simulink model "project"  (R2017b)
settings: Solver=FixedStepDiscrete  StartTime=0.0  StopTime=inf  RelTol=1e-3
PreLoadFcn:
  | load('commwlan80211BusTypes')
PostLoadFcn:
  | commwlan80211BeaconModelParams('init')
InitFcn:
  | load('commwlan80211BusTypes')
model workspace: external: MAT-File (data not in the file)
undefined symbols (not defined in the file): commwlan80211TxFilt, p80211
libraries: commutil2 x6, commwlan80211BeaconLib x6, commcrc2 x3, commdigbbndpm3 x2, commsequence2 x2, commfilt2 x2, simulink x1, commsync2 x1, dspsigops x1, commchan3 x1, commrflib2 x1, commblksprivate x1
CloseFcn:
  | hFig = findall(0, 'Type', 'figure', 'Name', '802.11 Beacon Frame');
  | if ishghandle(hFig)
  | close(hFig);
  | end
  | clear hFig
Description:
  | IEEE 802.11 WLAN Beacon Frame
settings Model: Creator=The MathWorks, Inc.  LastModifiedBy=Josh Andrews
settings DataIOCC: LimitDataPoints=on  SaveFormat=Array  SaveOutput=off  SignalLogging=off  SaveTime=off
settings OptimizationCC: ExpressionDepthLimit=2147483647  LifeSpan=inf
settings DebuggingCC: UnderspecifiedInitializationDetection=Classic  MergeDetectMultiDrivingBlocksExec=none  SolverPrmCheckMsg=warning  FcnCallInpInsideContextMsg=warning  UniqueDataStoreMsg=error  AllowSymbolicDim=off  StateNameClashWarn=warning  SFUnexpectedBacktrackingDiag=warning  SFNoUnconditionalDefaultTransitionDiag=warning  SFExecutionAtInitializationDiag=none
settings HardwareCC: ProdBitPerPointer=32  ProdBitPerSizeT=32  ProdBitPerPtrDiffT=32  ProdLargestAtomicFloat=None  ProdIntDivRoundTo=Undefined  ProdEndianess=Unspecified  ProdWordSize=32  ProdHWDeviceType=32-bit Generic
settings ModelReferenceCC: PropagateSignalLabelsOutOfModel=off
settings CodeAppCC: StateflowObjectComments=on
settings GRTTargetCC: TargetLangStandard=C89/C90 (ANSI)  GeneratePreprocessorConditionals=Disable all  CombineOutputUpdateFcns=off  GRTInterface=on
settings ConfigComp: CovMetricSettings=dw  CovHtmlReporting=on  CovSaveCumulativeToWorkspaceVar=on  CovSaveSingleToWorkspaceVar=on  CovExternalEMLEnable=off  CovSFcnEnable=off

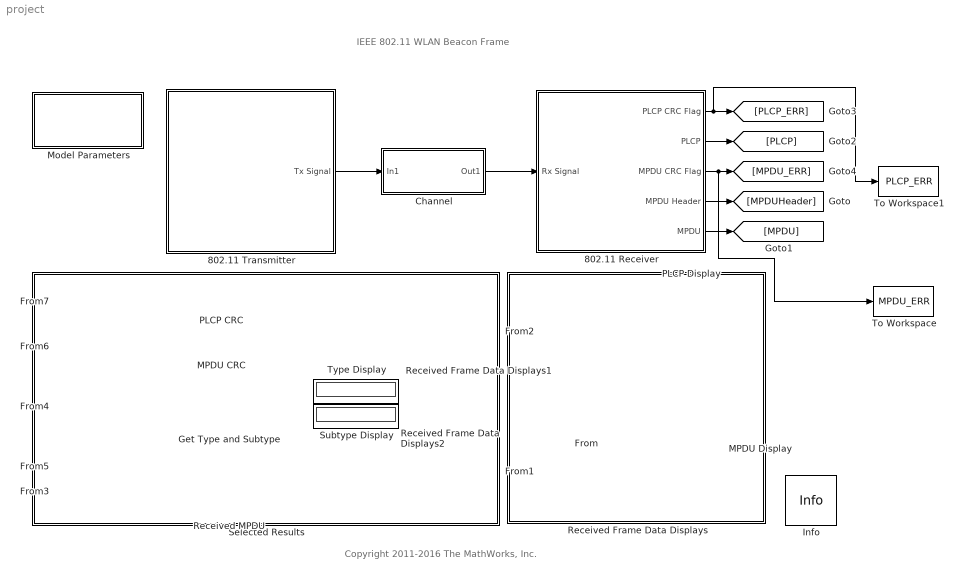
== system project ==
  note: IEEE 802.11 WLAN
      | Beacon Frame
  note: Copyright 2011-2016 The MathWorks, Inc.
  802.11 Receiver : Subsystem
  802.11 Transmitter : Subsystem
  Channel : Subsystem  BlockChoice=Delay only  mask(Channel){EsNo=0, freqOffset=100, delay=1e-06}
      mask prompts: EsNo "EsNo (dB):"; freqOffset "Frequency offset (Hz):"; delay "Delay (s):"
      mask help: Choose the channel type.
      settings: AttributesFormatString=Es/No = %<EsNo> dB\nFrequency offset = %<freqOffset> Hz\nDelay = %<delay> s
      mask Display: disp('Channel');
  Get Type and Subtype : Subsystem
  Info : commblksprivate/Info  SystemSampleTime=-1
      settings: SourceProductName=Communications System Toolbox  SourceProductBaseCode=CM
  MPDU CRC : Display
  MPDU Display : Subsystem
  Model Parameters : Subsystem  mask(Model Parameters){paramSet=Beacon frame parameters, beaconInterval=2, ssidValue='MathWorks SDR team', rates=[1 2 5], channelNumber=1, sendCFParams=on, cfpCount=2, cfpPeriod=5, cfpMaxDuration=10, cfpDurRemain=5, EsNo=0, freqOffset=100, delay=1e-6}
      mask prompts: paramSet "Parameter set:"; beaconInterval "Beacon interval (TU):"; ssidValue "SSID value:"; rates "Supported rates (Mbps):"; channelNumber "Channel number:"; sendCFParams "Send CF Parameters set element"; cfpCount "CFP Count (DTIM intervals):"; cfpPeriod "CFP Period (DTIM intervals):"; cfpMaxDuration "CFP MaxDuration (TU):"; cfpDurRemain "CFP DurRemaining (TU):"; EsNo "Es/No (dB):"; freqOffset "Frequency offset (Hz):"; delay "Delay (s):"
      mask help:
      | Choose beacon frame parameters and channel parameters.
      |
      | When you select the parameter set as 'Beacon frame parameters', you can set SSID, beacon interval, supported rates, channel number. You can also optionally send CF parameters set element in the beacon frame. The 'Beacon interval (TU)' parameter sets the period of beacon transmissions in time units (TU), which is 1024 microseconds.
      |
      | When you select the parameter set as 'Channel parameters', you can set noise level, frequency offset, and delay the channel introduces.
      mask init:
      | commwlan80211BeaconModelParams('init')
      settings: AttributesFormatString=Beacon interval = %<beaconInterval> TU
      mask Help: helpview(commdhelp);
      mask TypeOptions paramSet: Beacon frame parameters | Channel parameters
      mask Callback paramSet: commwlan80211BeaconModelParams('cbParamSet');
      mask TypeOptions channelNumber: 1 | 2 | 3 | 4 | 5 | 6 | 7 | 8 | 9 | 10 | 11
      mask Callback sendCFParams: commwlan80211BeaconModelParams('cbSendCFParams');
      mask Display: disp('Model\nParameters')
  PLCP CRC : Display
  PLCP Display : Subsystem
  Received Frame Data Displays : Subsystem
      mask Display: disp('')
  Received Frame Data Displays1 : Subsystem
      mask Display: disp('0 = Management')
  Received Frame Data Displays2 : Subsystem
      mask Display: disp('8 = Beacon')
  Received MPDU : Subsystem  mask(Received MPDU GUI){OpenScopeAtSimStart=on, openGUIBoolean=true}
      mask prompts: OpenScopeAtSimStart "Open GUI at start of simulation"; openGUIBoolean "Open GUI Boolean"
      mask help: Show selected information from the received Beacon frame.
      mask Callback OpenScopeAtSimStart:
      | if strcmp(get_param(gcb,'OpenScopeAtSimStart'), 'on')
      |   set_param(gcb,'openGUIBoolean','true');
      | else
      |   set_param(gcb,'openGUIBoolean','false');
      | end
      mask Display: disp('MPDU GUI')
  Selected Results : Subsystem
      mask Display: disp('')
  Subtype Display : Display
  To Workspace : ToWorkspace  VariableName=MPDU_ERR  SaveFormat=Timeseries  SampleTime=-1
  To Workspace1 : ToWorkspace  VariableName=PLCP_ERR  SaveFormat=Timeseries  SampleTime=-1
  Type Display : Display
  wires:
  Channel/1(Out1) -> 802.11 Receiver/1(Rx Signal)
  802.11 Receiver/1(PLCP CRC Flag) -> To Workspace1/1, [PLCP_ERR]
  802.11 Receiver/3(MPDU CRC Flag) -> To Workspace/1, [MPDU_ERR]
  802.11 Receiver/4(MPDU Header) -> [MPDUHeader]
  802.11 Receiver/5(MPDU) -> [MPDU]
  802.11 Receiver/2(PLCP) -> [PLCP]
  [MPDUHeader] -> MPDU Display/1(Header)
  [MPDU] -> MPDU Display/2(Payload)
  802.11 Transmitter/1(Tx Signal) -> Channel/1(In1)
  [PLCP] -> PLCP Display/1(PLCP)
  [MPDUHeader] -> Get Type and Subtype/1(In1)
  Get Type and Subtype/1(Type) -> Type Display/1
  Get Type and Subtype/2(Subtype) -> Subtype Display/1
  [MPDU] -> Received MPDU/2(mpdu)
  [MPDU_ERR] -> MPDU CRC/1
  [PLCP_ERR] -> PLCP CRC/1
  [MPDU_ERR] -> Received MPDU/1(trigger)

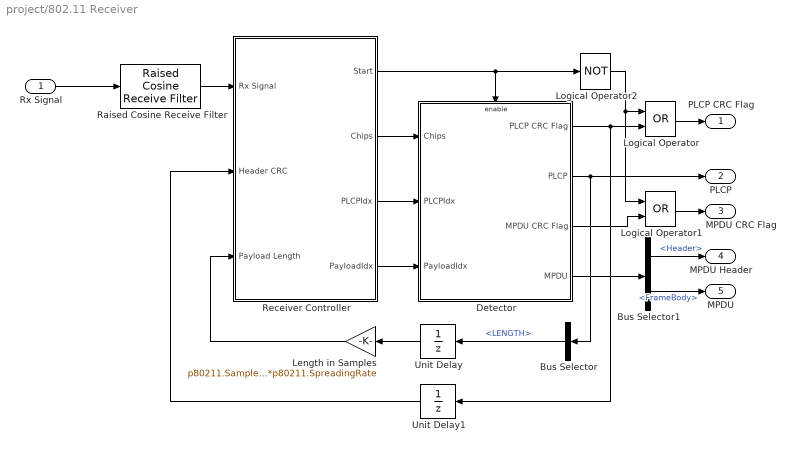
== system project/802.11 Receiver ==
  Rx Signal : Inport
  Bus Selector : BusSelector  OutputSignals=LENGTH
  Bus Selector1 : BusSelector  OutputSignals=Header,FrameBody
  Detector : Subsystem
  Length in Samples : Gain  Gain=p80211.SamplesPerChip*p80211.SpreadingRate  OutDataTypeStr=uint32  SaturateOnIntegerOverflow=on  ParamDataTypeStr=Inherit: Same as input
  Logical Operator : Logic  Operator=OR  AllPortsSameDT=off  OutDataTypeStr=boolean
  Logical Operator1 : Logic  Operator=OR  AllPortsSameDT=off  OutDataTypeStr=boolean
  Logical Operator2 : Logic  Operator=NOT  AllPortsSameDT=off  OutDataTypeStr=boolean
  Raised Cosine Receive Filter : commfilt2/Raised Cosine Receive Filter  filtType=Square root  R=0.3  filtSpan=p80211.FilterOrder  N=p80211.SamplesPerChip  downFactor=1  downOffset=0  filterGain=1  InputProcessing=Columns as channels (frame based)  RateOptions=Enforce single-rate processing  framing=Mute  checkCoeff=off  variableName=rcRxFilt  currentFiltSpan=2*(p80211.FilterOrder/2)  D=p80211.FilterOrder/2  inputOffset=0  sampMode=Mute  saveAsFlag=0  rateMode=Downsampling  checkGain=Normalized  launchFVT=off  roundingMode=Floor  overflowMode=off  coeffDataTypeStr=Inherit: Same word length as input  coeffMin=[]  coeffMax=[]  coeffLastDataTypeStr=Inherit: Same word length as input  accumDataTypeStr=Inherit: Same as product output  accumLastDataTypeStr=Inherit: Same as product output  outputDataTypeStr=Inherit: Same as accumulator  outputMin=[]  outputMax=[]  outputLastDataTypeStr=Inherit: Same as accumulator
  Receiver Controller : Subsystem
  Unit Delay : UnitDelay  InitialCondition=p80211.SymbolsPerChannelFrame  SampleTime=-1
  Unit Delay1 : UnitDelay  InitialCondition=1  SampleTime=-1
  PLCP CRC Flag : Outport
  PLCP : Outport  Port=2
  MPDU CRC Flag : Outport  Port=3
  MPDU Header : Outport  Port=4
  MPDU : Outport  Port=5
  wires:
  Raised Cosine Receive Filter/1 -> Receiver Controller/1(Rx Signal)
  Receiver Controller/2(Chips) -> Detector/1(Chips)
  Receiver Controller/1(Start) -> Detector/Enable, Logical Operator2/1
  Receiver Controller/3(PLCPIdx) -> Detector/2(PLCPIdx)
  Receiver Controller/4(PayloadIdx) -> Detector/3(PayloadIdx)
  Unit Delay/1 -> Length in Samples/1
  Length in Samples/1 -> Receiver Controller/3(Payload Length)
  Rx Signal/1 -> Raised Cosine Receive Filter/1
  Detector/1(PLCP CRC Flag) -> Logical Operator/2, Unit Delay1/1
  Detector/2(PLCP) -> PLCP/1, Bus Selector/1
  Unit Delay1/1 -> Receiver Controller/2(Header CRC)
  Bus Selector/1 -> Unit Delay/1  "<LENGTH>"
  Logical Operator/1 -> PLCP CRC Flag/1
  Logical Operator1/1 -> MPDU CRC Flag/1
  Detector/3(MPDU CRC Flag) -> Logical Operator1/2
  Logical Operator2/1 -> Logical Operator/1, Logical Operator1/1
  Detector/4(MPDU) -> Bus Selector1/1
  Bus Selector1/1 -> MPDU Header/1  "<Header>"
  Bus Selector1/2 -> MPDU/1  "<FrameBody>"

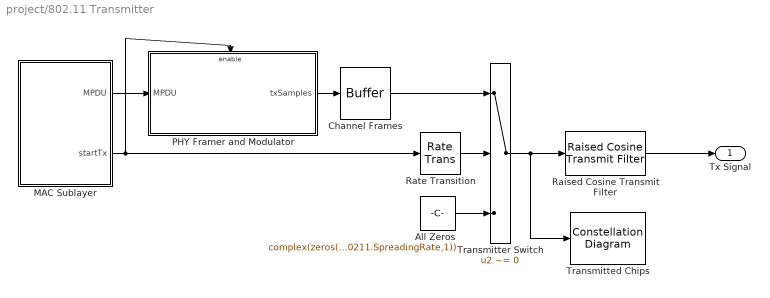
== system project/802.11 Transmitter ==
  All Zeros : Constant  Value=complex(zeros(p80211.SymbolsPerChannelFrame*p80211.SpreadingRate,1))  VectorParams1D=off
  Channel Frames : Buffer  N=p80211.SymbolsPerChannelFrame*p80211.SpreadingRate  OutputFrames=off
  MAC Sublayer : Subsystem
  PHY Framer and Modulator : Subsystem
  Raised Cosine Transmit Filter : commfilt2/Raised Cosine Transmit Filter  filtType=Square root  R=0.3  filtSpan=p80211.FilterOrder  N=p80211.SamplesPerChip  filterGain=1  InputProcessing=Columns as channels (frame based)  RateOptions=Enforce single-rate processing  framing=Mute  checkCoeff=on  variableName=commwlan80211TxFilt  checkGain=Normalized  sampMode=Mute  saveAsFlag=0  currentFiltSpan=2*(p80211.FilterOrder/2)  D=p80211.FilterOrder/2  launchFVT=off  roundingMode=Floor  overflowMode=off  coeffDataTypeStr=Inherit: Same word length as input  coeffMin=[]  coeffMax=[]  coeffLastDataTypeStr=Inherit: Same word length as input  outputDataTypeStr=Inherit: Same as accumulator  outputMin=[]  outputMax=[]  outputLastDataTypeStr=Inherit: Same as accumulator
  Rate Transition : RateTransition
  Transmitted Chips : ConstellationDiagram  Tag=ScatterPlot
  Transmitter Switch : Switch  Criteria=u2 ~= 0
  Tx Signal : Outport
  wires:
  PHY Framer and Modulator/1(txSamples) -> Channel Frames/1
  All Zeros/1 -> Transmitter Switch/3
  Transmitter Switch/1 -> Transmitted Chips/1, Raised Cosine Transmit Filter/1
  MAC Sublayer/2(startTx) -> PHY Framer and Modulator/Enable, Rate Transition/1
  Channel Frames/1 -> Transmitter Switch/1
  MAC Sublayer/1(MPDU) -> PHY Framer and Modulator/1(MPDU)
  Raised Cosine Transmit Filter/1 -> Tx Signal/1
  Rate Transition/1 -> Transmitter Switch/2

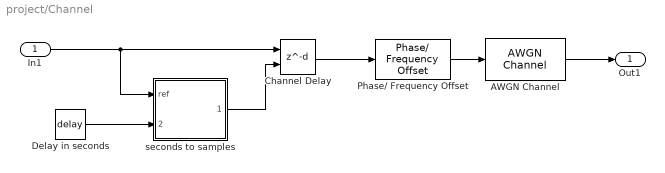
== system project/Channel ==
  In1 : Inport
  AWGN Channel : commchan3/AWGN Channel  InputProcessing=Columns as channels (frame based)  seed=1237  noiseMode="Signal to noise ratio  (Es/No)"  EbNodB=10  EsNodB=EsNo  SNRdB=10  bitsPerSym=1  Ps=sum(commwlan80211TxFilt.^2)/p80211.SamplesPerChip  Tsym=1/p80211.ChipRate  variance=1
  Channel Delay : Delay  DelayLengthSource=Input port  DelayLength=10  DelayLengthUpperLimit=1024e-6*p80211.ChipRate*p80211.SamplesPerChip  InputProcessing=Columns as channels (frame based)
      settings: InputPortMap=u0,p1
  Delay in seconds : Constant  Value=delay
  Phase/ Frequency Offset : commrflib2/Phase// Frequency Offset  phaseOffset=0  freqPort=off  freqOffset=freqOffset
      settings: SourceProductName=Communications System Toolbox
  seconds to samples : Subsystem
  Out1 : Outport
  wires:
  In1/1 -> Channel Delay/1, seconds to samples/1(ref)
  Channel Delay/1 -> Phase/ Frequency Offset/1
  AWGN Channel/1 -> Out1/1
  Phase/ Frequency Offset/1 -> AWGN Channel/1
  Delay in seconds/1 -> seconds to samples/2(seconds)
  seconds to samples/1(samples) -> Channel Delay/2

== system project/Get Type and Subtype ==
  In1 : Inport
  Bus Selector3 : BusSelector  OutputSignals=FrameCtrl.Type,FrameCtrl.Subtype
  Type : Outport
  Subtype : Outport  Port=2
  wires:
  Bus Selector3/1 -> Type/1  "<Type>"
  In1/1 -> Bus Selector3/1
  Bus Selector3/2 -> Subtype/1  "<Subtype>"

== system project/MPDU Display ==
  Header : Inport
  Payload : Inport  Port=2
  MAC Header Display : Subsystem
  MAC Payload Display : Subsystem
  wires:
  Header/1 -> MAC Header Display/1(Header)
  Payload/1 -> MAC Payload Display/1(Payload)

== system project/Model Parameters ==

== system project/PLCP Display ==
  note: IEEE 802.11
      | PLCP Contents
  PLCP : Inport
  Bus Selector5 : BusSelector  OutputSignals=SFD,SIGNAL,SERVICE,LENGTH
  LENGTH Display : Display
  SERVICE Display : Display
      settings: Format=hex (Stored Integer)
  SFD Display : Display
      settings: Format=hex (Stored Integer)
  SIGNAL Display : Display
      settings: Format=hex (Stored Integer)
  wires:
  PLCP/1 -> Bus Selector5/1
  Bus Selector5/4 -> LENGTH Display/1  "<LENGTH>"
  Bus Selector5/1 -> SFD Display/1  "<SFD>"
  Bus Selector5/2 -> SIGNAL Display/1  "<SIGNAL>"
  Bus Selector5/3 -> SERVICE Display/1  "<SERVICE>"

== system project/Received Frame Data Displays ==

== system project/Received Frame Data Displays1 ==

== system project/Received Frame Data Displays2 ==

== system project/Received MPDU ==
  trigger : Inport
  mpdu : Inport  Port=2
  Logical Operator2 : Logic  Operator=NOT  AllPortsSameDT=off  OutDataTypeStr=boolean
  Received MPDU GUI : MATLAB Function  TreatAsAtomicUnit=on
  wires:
  trigger/1 -> Logical Operator2/1
  mpdu/1 -> Received MPDU GUI/1(mpdu)
  Logical Operator2/1 -> Received MPDU GUI/Trigger

== system project/Selected Results ==

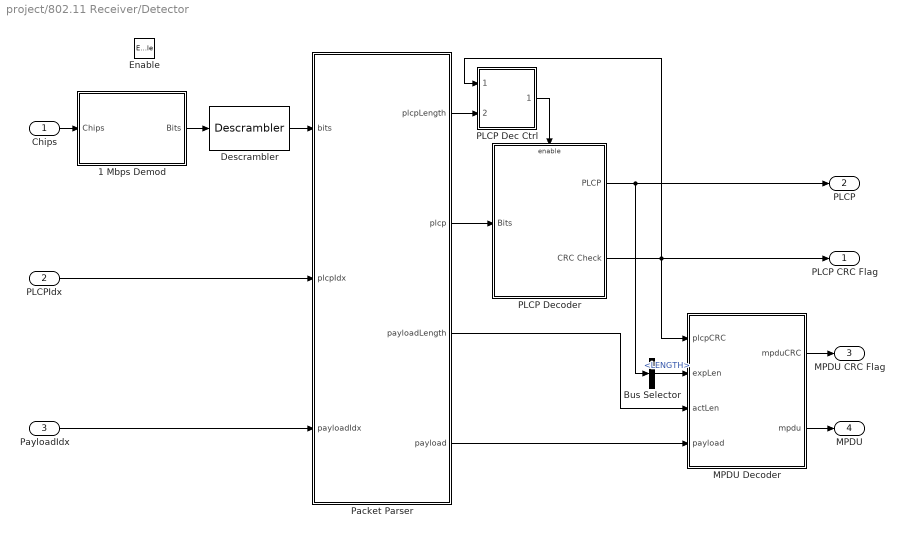
== system project/802.11 Receiver/Detector ==
  Chips : Inport
  PLCPIdx : Inport  Port=2
  PayloadIdx : Inport  Port=3
  Enable : EnablePort  StatesWhenEnabling=reset  PropagateVarSize=During execution
  1 Mbps Demod : Subsystem
  Bus Selector : BusSelector  OutputSignals=LENGTH
  Descrambler : commsequence2/Descrambler  M=2  poly=p80211.ScramblerPolynomial  iniStaSource=Dialog Parameter  ini_sta=[0 0 0 0 0 0 0]  resetViaPort=off
      settings: SourceProductName=Communications System Toolbox  SourceProductBaseCode=CM
  MPDU Decoder : MATLAB Function  TreatAsAtomicUnit=on
  PLCP Dec Ctrl : Subsystem
  PLCP Decoder : Subsystem
  Packet Parser : MATLAB Function  TreatAsAtomicUnit=on
  PLCP CRC Flag : Outport  InitialOutput=1
  PLCP : Outport  Port=2
  MPDU CRC Flag : Outport  Port=3  InitialOutput=1
  MPDU : Outport  Port=4
  wires:
  1 Mbps Demod/1(Bits) -> Descrambler/1
  Chips/1 -> 1 Mbps Demod/1(Chips)
  PLCP Decoder/2(CRC Check) -> PLCP CRC Flag/1, PLCP Dec Ctrl/1(CRC Flag), MPDU Decoder/1(plcpCRC)
  MPDU Decoder/1(mpduCRC) -> MPDU CRC Flag/1
  PLCPIdx/1 -> Packet Parser/2(plcpIdx)
  PayloadIdx/1 -> Packet Parser/3(payloadIdx)
  Packet Parser/2(plcp) -> PLCP Decoder/1(Bits)
  Packet Parser/1(plcpLength) -> PLCP Dec Ctrl/2(Length)
  Packet Parser/4(payload) -> MPDU Decoder/4(payload)
  Descrambler/1 -> Packet Parser/1(bits)
  MPDU Decoder/2(mpdu) -> MPDU/1
  PLCP Decoder/1(PLCP) -> PLCP/1, Bus Selector/1
  Bus Selector/1 -> MPDU Decoder/2(expLen)  "<LENGTH>"
  PLCP Dec Ctrl/1(Enable) -> PLCP Decoder/Enable
  Packet Parser/3(payloadLength) -> MPDU Decoder/3(actLen)

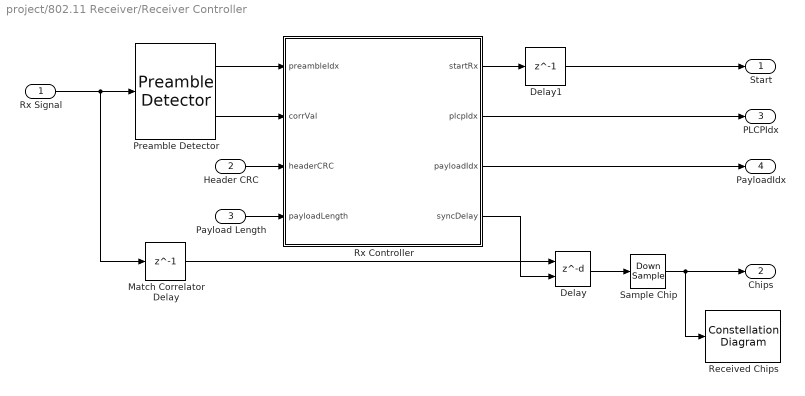
== system project/802.11 Receiver/Receiver Controller ==
  Rx Signal : Inport
  Header CRC : Inport  Port=2
  Payload Length : Inport  Port=3
  Delay : Delay  DelayLengthSource=Input port  DelayLengthUpperLimit=11264  InputProcessing=Columns as channels (frame based)
      settings: InputPortMap=u0,p1
  Delay1 : Delay  DelayLength=1  InitialCondition=0  UseCircularBuffer=on
  Match Correlator Delay : Delay  DelayLength=1  InitialCondition=0  UseCircularBuffer=on
  Preamble Detector : commsync2/Preamble Detector  Input=Symbol  Preamble=p80211.SynchronizationSignal  Threshold=p80211.CorrelationThreshold  DetectionMetricOutput=on  Detections=All  SimulateUsing=Interpreted execution
      settings: SourceProductName=Communications System Toolbox  SourceProductBaseCode=CM
  Received Chips : ConstellationDiagram  Tag=ScatterPlot
  Rx Controller : MATLAB Function  TreatAsAtomicUnit=on
  Sample Chip : DownSample  N=p80211.SamplesPerChip
  Start : Outport
  Chips : Outport  Port=2
  PLCPIdx : Outport  Port=3
  PayloadIdx : Outport  Port=4
  wires:
  Rx Signal/1 -> Match Correlator Delay/1, Preamble Detector/1
  Sample Chip/1 -> Chips/1, Received Chips/1
  Delay/1 -> Sample Chip/1
  Rx Controller/4(syncDelay) -> Delay/2
  Rx Controller/1(startRx) -> Delay1/1
  Delay1/1 -> Start/1
  Rx Controller/2(plcpIdx) -> PLCPIdx/1
  Rx Controller/3(payloadIdx) -> PayloadIdx/1
  Header CRC/1 -> Rx Controller/3(headerCRC)
  Match Correlator Delay/1 -> Delay/1
  Payload Length/1 -> Rx Controller/4(payloadLength)
  Preamble Detector/1 -> Rx Controller/1(preambleIdx)
  Preamble Detector/2 -> Rx Controller/2(corrVal)

== system project/802.11 Transmitter/MAC Sublayer ==
  FCS : Subsystem
  MPDU Indices : Constant  Value=(1:p80211.NumMPDUOctets)'  VectorParams1D=off
  Selector : Selector  IndexOptions=Index vector (port)  Indices=[1:p80211.NumMPDUOctets]  OutputSizes=1
  Transmitter Controller : MATLAB Function  TreatAsAtomicUnit=on
  MPDU : Outport
  startTx : Outport  Port=2
  wires:
  Transmitter Controller/2(startTx) -> startTx/1
  FCS/1(Out1) -> MPDU/1
  MPDU Indices/1 -> Selector/2
  Selector/1 -> FCS/1(In1)
  Transmitter Controller/1(payload) -> Selector/1

== system project/802.11 Transmitter/PHY Framer and Modulator ==
  note: Reference: IEEE Std 802.11 - 2007, Section 15.2.4
  MPDU : Inport
  Enable : EnablePort  StatesWhenEnabling=reset
  1 Mbps Mod : Subsystem
  1024 Framer : dspsigops/Pad  padAlong=Columns  dimsToPad=1  valSrc=Specify via dialog  padVal=0  spec=Output size  padNumOutRowsSpecMethod=User-specified  numOutRows=p80211.MaximumPPDULength*p80211.SpreadingRate  padNumOutColsSpecMethod=User-specified  numOutCols=1  isVarDimsMode=off  padBeginning=0  padEnd=0  outSizeMode=User-specified  outSize=1  padSigAt=End  trunc_flag=None  roundingMode=Floor  overflowMode=off  truncOrWrapMode=Truncate  wrap_flag=None
      settings: SourceProductName=DSP System Toolbox  SourceProductBaseCode=DS
  Framing by adding PLCP preamble and header : Subsystem
  Scrambler z^-7+z^-4+1 : commsequence2/Scrambler  M=2  poly=p80211.ScramblerPolynomial  iniStaSource=Dialog Parameter  ini_sta=[0 0 0 0 0 0 0]  resetViaPort=off
      settings: SourceProductName=Communications System Toolbox  SourceProductBaseCode=CM
  txSamples : Outport
  wires:
  Framing by adding PLCP preamble and header/1(PPDU) -> Scrambler z^-7+z^-4+1/1
  1 Mbps Mod/1(Out1) -> 1024 Framer/1
  1024 Framer/1 -> txSamples/1
  MPDU/1 -> Framing by adding PLCP preamble and header/1(MPDU)
  Scrambler z^-7+z^-4+1/1 -> 1 Mbps Mod/1(In1)

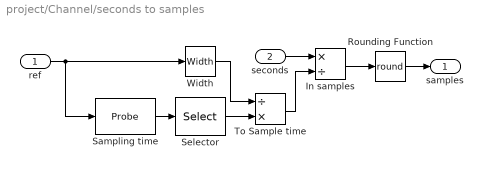
== system project/Channel/seconds to samples ==
  ref : Inport
  seconds : Inport  Port=2
  In samples : Product  Inputs=*/
  Rounding Function : Rounding  Operator=round
  Sampling time : Probe  ProbeWidth=off  ProbeComplexSignal=off
  Selector : Selector  InputPortWidth=2  IndexOptions=Index vector (dialog)  Indices=1  OutputSizes=1
  To Sample time : Product  Inputs=/*
  Width : Width
  samples : Outport
  wires:
  Sampling time/1 -> Selector/1
  In samples/1 -> Rounding Function/1
  Width/1 -> To Sample time/1
  Selector/1 -> To Sample time/2
  ref/1 -> Width/1, Sampling time/1
  Rounding Function/1 -> samples/1
  seconds/1 -> In samples/1
  To Sample time/1 -> In samples/2

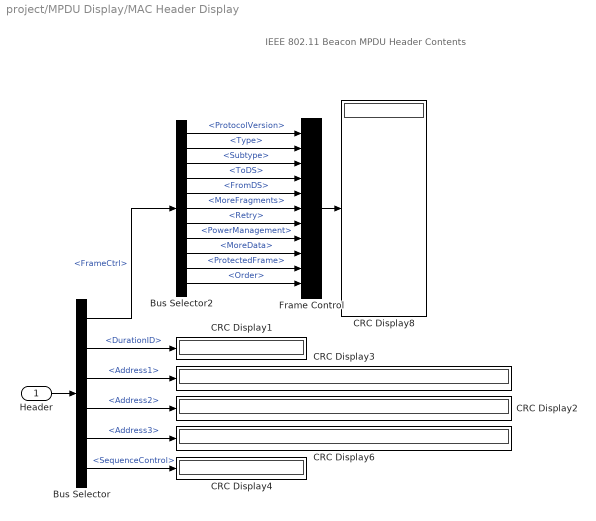
== system project/MPDU Display/MAC Header Display ==
  note: IEEE 802.11
      |   Beacon MPDU Header Contents
  Header : Inport
  Bus Selector : BusSelector  OutputSignals=FrameCtrl,DurationID,Address1,Address2,Address3,SequenceControl
  Bus Selector2 : BusSelector  OutputSignals=ProtocolVersion,Type,Subtype,ToDS,FromDS,MoreFragments,Retry,PowerManagement,MoreData,ProtectedFrame,Order
  CRC Display{1..4,6,8} (6 alike) : Display
      CRC Display1 settings: Format=hex (Stored Integer)
      CRC Display2 settings: Format=hex (Stored Integer)
      CRC Display3 settings: Format=hex (Stored Integer)
      CRC Display4 settings: Format=hex (Stored Integer)
      CRC Display6 settings: Format=hex (Stored Integer)
  Frame Control : Concatenate  NumInputs=11  Mode=Multidimensional array
  wires:
  Bus Selector/2 -> CRC Display1/1  "<DurationID>"
  Bus Selector/3 -> CRC Display3/1  "<Address1>"
  Bus Selector/4 -> CRC Display2/1  "<Address2>"
  Bus Selector2/1 -> Frame Control/1  "<ProtocolVersion>"
  Bus Selector2/2 -> Frame Control/2  "<Type>"
  Bus Selector2/3 -> Frame Control/3  "<Subtype>"
  Bus Selector2/4 -> Frame Control/4  "<ToDS>"
  Bus Selector2/5 -> Frame Control/5  "<FromDS>"
  Bus Selector2/6 -> Frame Control/6  "<MoreFragments>"
  Bus Selector2/7 -> Frame Control/7  "<Retry>"
  Bus Selector2/8 -> Frame Control/8  "<PowerManagement>"
  Bus Selector2/9 -> Frame Control/9  "<MoreData>"
  Bus Selector2/10 -> Frame Control/10  "<ProtectedFrame>"
  Bus Selector2/11 -> Frame Control/11  "<Order>"
  Frame Control/1 -> CRC Display8/1
  Bus Selector/5 -> CRC Display6/1  "<Address3>"
  Bus Selector/6 -> CRC Display4/1  "<SequenceControl>"
  Header/1 -> Bus Selector/1
  Bus Selector/1 -> Bus Selector2/1  "<FrameCtrl>"

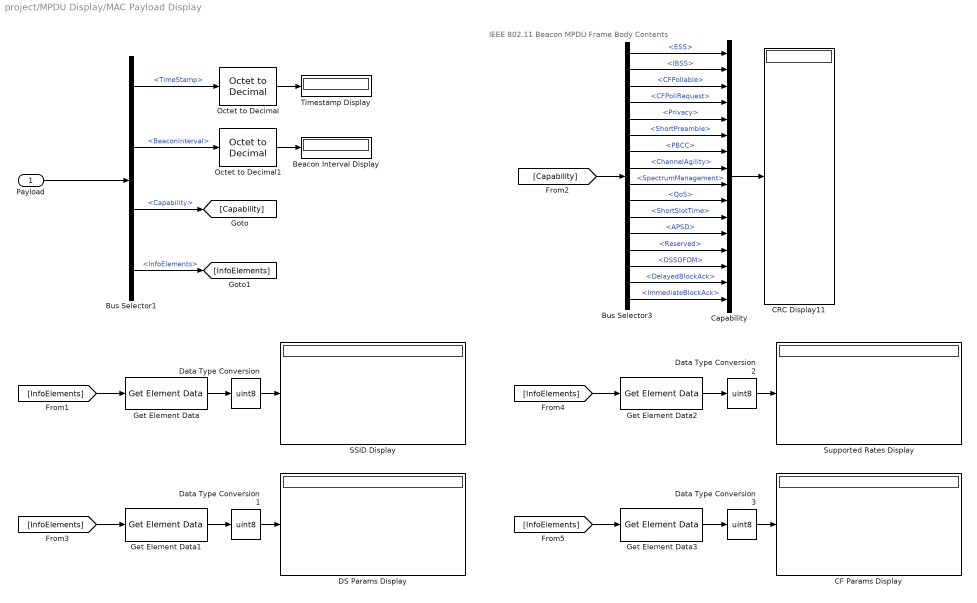
== system project/MPDU Display/MAC Payload Display ==
  note: IEEE 802.11
      |   Beacon MPDU Frame Body Contents
  Payload : Inport
  Beacon Interval Display : Display
  Bus Selector1 : BusSelector  OutputSignals=TimeStamp,BeaconInterval,Capability,InfoElements
  Bus Selector3 : BusSelector  OutputSignals=ESS,IBSS,CFPollable,CFPollRequest,Privacy,ShortPreamble,PBCC,ChannelAgility,SpectrumManagement,QoS,ShortSlotTime,APSD,Reserved,DSSOFDM,DelayedBlockAck,ImmediateBlockAck
  CF Params Display : Display
      settings: Format=hex (Stored Integer)
  CRC Display11 : Display
  Capability : Concatenate  NumInputs=16  Mode=Multidimensional array
  DS Params Display : Display
      settings: Format=hex (Stored Integer)
  Data Type Conversion{,1..3} (4 alike) : DataTypeConversion  OutDataTypeStr=uint8
  Get Element Data : commwlan80211BeaconLib/Get Element Data  elemIDIdx=SSID
      settings: SourceProductName=Communications System Toolbox  SourceProductBaseCode=CM
  Get Element Data1 : commwlan80211BeaconLib/Get Element Data  elemIDIdx=DS Parameters
      settings: SourceProductName=Communications System Toolbox  SourceProductBaseCode=CM
  Get Element Data2 : commwlan80211BeaconLib/Get Element Data  elemIDIdx=Supported Rates
      settings: SourceProductName=Communications System Toolbox  SourceProductBaseCode=CM
  Get Element Data3 : commwlan80211BeaconLib/Get Element Data  elemIDIdx=CF Parameters
      settings: SourceProductName=Communications System Toolbox  SourceProductBaseCode=CM
  Octet to Decimal : commwlan80211BeaconLib/Octet to Decimal
      settings: SourceProductName=Communications System Toolbox  SourceProductBaseCode=CM
  Octet to Decimal1 : commwlan80211BeaconLib/Octet to Decimal
      settings: SourceProductName=Communications System Toolbox  SourceProductBaseCode=CM
  SSID Display : Display
      settings: Format=hex (Stored Integer)
  Supported Rates Display : Display
      settings: Format=hex (Stored Integer)
  Timestamp Display : Display
  wires:
  Data Type Conversion1/1 -> DS Params Display/1
  Data Type Conversion2/1 -> Supported Rates Display/1
  Data Type Conversion3/1 -> CF Params Display/1
  [InfoElements] -> Get Element Data3/1
  Get Element Data3/1 -> Data Type Conversion3/1
  [InfoElements] -> Get Element Data2/1
  Get Element Data2/1 -> Data Type Conversion2/1
  [InfoElements] -> Get Element Data1/1
  Get Element Data1/1 -> Data Type Conversion1/1
  Data Type Conversion/1 -> SSID Display/1
  [InfoElements] -> Get Element Data/1
  Bus Selector3/11 -> Capability/11  "<ShortSlotTime>"
  Bus Selector1/4 -> [InfoElements]  "<InfoElements>"
  Octet to Decimal/1 -> Timestamp Display/1
  [Capability] -> Bus Selector3/1
  Bus Selector1/3 -> [Capability]  "<Capability>"
  Get Element Data/1 -> Data Type Conversion/1
  Payload/1 -> Bus Selector1/1
  Capability/1 -> CRC Display11/1
  Bus Selector3/16 -> Capability/16  "<ImmediateBlockAck>"
  Bus Selector3/15 -> Capability/15  "<DelayedBlockAck>"
  Bus Selector3/14 -> Capability/14  "<DSSOFDM>"
  Bus Selector3/13 -> Capability/13  "<Reserved>"
  Bus Selector3/12 -> Capability/12  "<APSD>"
  Bus Selector3/10 -> Capability/10  "<QoS>"
  Bus Selector3/9 -> Capability/9  "<SpectrumManagement>"
  Bus Selector3/8 -> Capability/8  "<ChannelAgility>"
  Bus Selector3/7 -> Capability/7  "<PBCC>"
  Bus Selector3/6 -> Capability/6  "<ShortPreamble>"
  Bus Selector3/5 -> Capability/5  "<Privacy>"
  Bus Selector3/4 -> Capability/4  "<CFPollRequest>"
  Bus Selector3/3 -> Capability/3  "<CFPollable>"
  Bus Selector3/2 -> Capability/2  "<IBSS>"
  Bus Selector3/1 -> Capability/1  "<ESS>"
  Bus Selector1/2 -> Octet to Decimal1/1  "<BeaconInterval>"
  Bus Selector1/1 -> Octet to Decimal/1  "<TimeStamp>"
  Octet to Decimal1/1 -> Beacon Interval Display/1

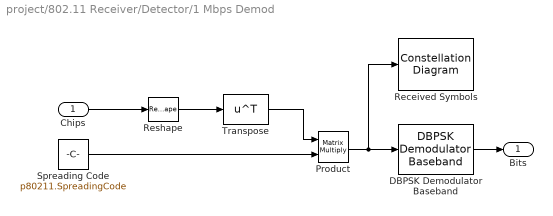
== system project/802.11 Receiver/Detector/1 Mbps Demod ==
  Chips : Inport
  DBPSK Demodulator Baseband : commdigbbndpm3/DBPSK Demodulator Baseband  Ph=0  outDtype=boolean
      settings: SourceProductName=Communications System Toolbox  SourceProductBaseCode=CM
  Product : Product  Multiplication=Matrix(*)  RndMeth=Zero
  Received Symbols : ConstellationDiagram  Tag=ScatterPlot
  Reshape : Reshape  OutputDimensionality=Customize  OutputDimensions=[length(p80211.SpreadingCode), p80211.SymbolsPerChannelFrame]
  Spreading Code : Constant  Value=p80211.SpreadingCode  VectorParams1D=off
  Transpose : Math  Operator=transpose  SaturateOnIntegerOverflow=on
  Bits : Outport
  wires:
  Product/1 -> DBPSK Demodulator Baseband/1, Received Symbols/1
  DBPSK Demodulator Baseband/1 -> Bits/1
  Reshape/1 -> Transpose/1
  Chips/1 -> Reshape/1
  Transpose/1 -> Product/1
  Spreading Code/1 -> Product/2

== system project/802.11 Receiver/Detector/PLCP Dec Ctrl ==
  note: After CRC decodes correctly (i.e. CRC Flag is 0)
      | disable the PLCP Decoder
  CRC Flag : Inport
  Length : Inport  Port=2
  Compare To Constant : simulink/Logic and Bit Operations/Compare To Constant  relop=>=  const=p80211.PLCPLength - length(p80211.SYNC)  OutDataTypeStr=uint8
  Logical Operator : Logic  AllPortsSameDT=off  OutDataTypeStr=boolean
  Unit Delay1 : UnitDelay  InitialCondition=1  SampleTime=-1
  Enable : Outport
  wires:
  Unit Delay1/1 -> Logical Operator/1
  CRC Flag/1 -> Unit Delay1/1
  Logical Operator/1 -> Enable/1
  Length/1 -> Compare To Constant/1
  Compare To Constant/1 -> Logical Operator/2

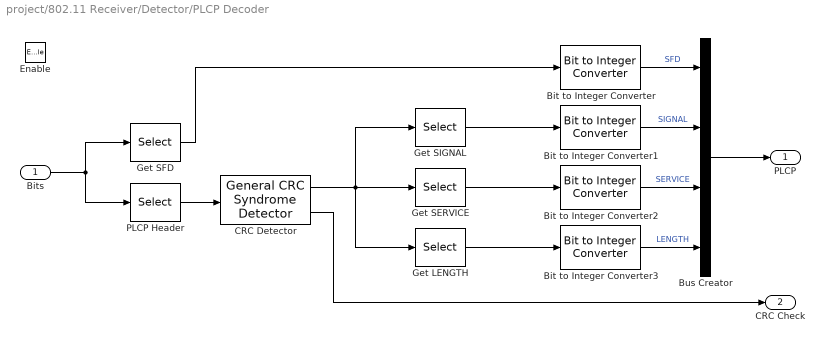
== system project/802.11 Receiver/Detector/PLCP Decoder ==
  Bits : Inport
  Enable : EnablePort  StatesWhenEnabling=reset  PropagateVarSize=During execution
  Bit to Integer Converter : commutil2/Bit to Integer Converter  nbits=16  bitOrder=LSB first  signedOutputValues=Unsigned  outDtype=Inherit via internal rule  outDtypeSigned=Inherit via internal rule
  Bit to Integer Converter1 : commutil2/Bit to Integer Converter  nbits=8  bitOrder=LSB first  signedOutputValues=Unsigned  outDtype=Inherit via internal rule  outDtypeSigned=Inherit via internal rule
  Bit to Integer Converter2 : commutil2/Bit to Integer Converter  nbits=8  bitOrder=LSB first  signedOutputValues=Unsigned  outDtype=Inherit via internal rule  outDtypeSigned=Inherit via internal rule
  Bit to Integer Converter3 : commutil2/Bit to Integer Converter  nbits=16  bitOrder=LSB first  signedOutputValues=Unsigned  outDtype=uint16  outDtypeSigned=Inherit via internal rule
  Bus Creator : BusCreator  Inputs=4
  CRC Detector : commcrc2/General CRC Syndrome Detector  genPoly=[1 0 0 0 1 0 0 0 0 0 0 1 0 0 0 0 1]  iniStates=1  directMethod=on  reflectInputBytes=off  reflectChecksums=off  finalXOR=1  numChecksums=1
      settings: SourceProductName=Communications System Toolbox  SourceProductBaseCode=CM
  Get LENGTH : Selector  InputPortWidth=32  IndexOptions=Index vector (dialog)  Indices=17:32  OutputSizes=1
  Get SERVICE : Selector  InputPortWidth=32  IndexOptions=Index vector (dialog)  Indices=9:16  OutputSizes=1
  Get SFD : Selector  InputPortWidth=p80211.PLCPHeaderLength + length(p80211.SFD) + length(p80211.ScramblerPolynomial)  IndexOptions=Index vector (dialog)  Indices=(1:16)+length(p80211.ScramblerPolynomial)  OutputSizes=1
  Get SIGNAL : Selector  InputPortWidth=32  IndexOptions=Index vector (dialog)  Indices=1:8  OutputSizes=1
  PLCP Header : Selector  InputPortWidth=p80211.PLCPHeaderLength + length(p80211.SFD) + length(p80211.ScramblerPolynomial)  IndexOptions=Index vector (dialog)  Indices=(17:64)+length(p80211.ScramblerPolynomial)  OutputSizes=1
  PLCP : Outport
  CRC Check : Outport  Port=2
  wires:
  PLCP Header/1 -> CRC Detector/1
  CRC Detector/1 -> Get LENGTH/1, Get SIGNAL/1, Get SERVICE/1
  Get SFD/1 -> Bit to Integer Converter/1
  Get SIGNAL/1 -> Bit to Integer Converter1/1
  Get SERVICE/1 -> Bit to Integer Converter2/1
  Get LENGTH/1 -> Bit to Integer Converter3/1
  Bit to Integer Converter/1 -> Bus Creator/1  "SFD"
  Bit to Integer Converter1/1 -> Bus Creator/2  "SIGNAL"
  Bit to Integer Converter2/1 -> Bus Creator/3  "SERVICE"
  Bits/1 -> Get SFD/1, PLCP Header/1
  Bit to Integer Converter3/1 -> Bus Creator/4  "LENGTH"
  Bus Creator/1 -> PLCP/1
  CRC Detector/2 -> CRC Check/1

== system project/802.11 Transmitter/MAC Sublayer/FCS ==
  In1 : Inport
  Convert octets to bits : commutil2/Integer to Bit Converter  nbits=8  signedInputValues=Unsigned  bitOrder=LSB first  outDtype=boolean
  MPDU CRC : commcrc2/General CRC Generator  genPoly=[32 26 23 22 16 12 11 10 8 7 5 4 2 1 0]  iniStates=1  directMethod=on  reflectInputBytes=off  reflectChecksums=off  finalXOR=1  numChecksums=1
      settings: SourceProductName=Communications System Toolbox  SourceProductBaseCode=CM
  Out1 : Outport
  wires:
  Convert octets to bits/1 -> MPDU CRC/1
  In1/1 -> Convert octets to bits/1
  MPDU CRC/1 -> Out1/1

== system project/802.11 Transmitter/PHY Framer and Modulator/1 Mbps Mod ==
  note: Reference: IEEE Std 802.11 - 2007, Section 15.4.6.3 and 15.4.6.4
  In1 : Inport
  Column vector : Reshape  OutputDimensionality=Column vector (2-D)
  DBPSK Modulator Baseband1 : commdigbbndpm3/DBPSK Modulator Baseband  Ph=0  outDtype=double
      settings: SourceProductName=Communications System Toolbox  SourceProductBaseCode=CM
  Row vector : Reshape  OutputDimensionality=Row vector (2-D)
  Spread with Barker code : Gain  Gain=p80211.SpreadingCode  Multiplication=Matrix(K*u)  SaturateOnIntegerOverflow=on  OutDataTypeStr=Inherit: Same as input  ParamDataTypeStr=Inherit: Same as input
  Out1 : Outport
  wires:
  Row vector/1 -> Spread with Barker code/1
  Spread with Barker code/1 -> Column vector/1
  DBPSK Modulator Baseband1/1 -> Row vector/1
  In1/1 -> DBPSK Modulator Baseband1/1
  Column vector/1 -> Out1/1  "PPDU"

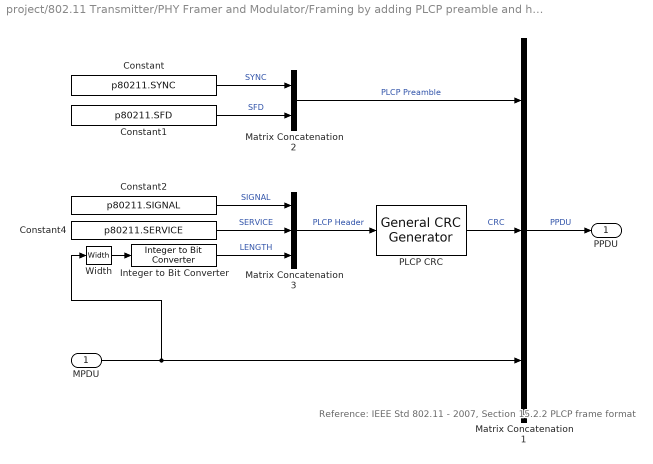
== system project/802.11 Transmitter/PHY Framer and Modulator/Framing by adding PLCP preamble and header ==
  note: Reference: IEEE Std 802.11 - 2007, Section 15.2.2 PLCP frame format
  MPDU : Inport
  Constant : Constant  Value=p80211.SYNC  VectorParams1D=off
  Constant1 : Constant  Value=p80211.SFD  VectorParams1D=off
  Constant2 : Constant  Value=p80211.SIGNAL  VectorParams1D=off
  Constant4 : Constant  Value=p80211.SERVICE  VectorParams1D=off
  Integer to Bit Converter : commutil2/Integer to Bit Converter  nbits=16  signedInputValues=Unsigned  bitOrder=LSB first  outDtype=boolean
  Matrix Concatenation1 : Concatenate  NumInputs=3  Mode=Multidimensional array
  Matrix Concatenation2 : Concatenate  Mode=Multidimensional array
  Matrix Concatenation3 : Concatenate  NumInputs=3  Mode=Multidimensional array
  PLCP CRC : commcrc2/General CRC Generator  genPoly=[1 0 0 0 1 0 0 0 0 0 0 1 0 0 0 0 1]  iniStates=1  directMethod=on  reflectInputBytes=off  reflectChecksums=off  finalXOR=1  numChecksums=1
      settings: SourceProductName=Communications System Toolbox  SourceProductBaseCode=CM
  Width : Width
  PPDU : Outport
  wires:
  Constant/1 -> Matrix Concatenation2/1  "SYNC"
  Matrix Concatenation2/1 -> Matrix Concatenation1/1  "PLCP Preamble"
  MPDU/1 -> Matrix Concatenation1/3, Width/1
  Matrix Concatenation1/1 -> PPDU/1  "PPDU"
  Width/1 -> Integer to Bit Converter/1
  Constant4/1 -> Matrix Concatenation3/2  "SERVICE"
  Constant2/1 -> Matrix Concatenation3/1  "SIGNAL"
  Constant1/1 -> Matrix Concatenation2/2  "SFD"
  Matrix Concatenation3/1 -> PLCP CRC/1  "PLCP Header"
  PLCP CRC/1 -> Matrix Concatenation1/2  "CRC"
  Integer to Bit Converter/1 -> Matrix Concatenation3/3  "LENGTH"

== matlab function project/Received MPDU/Received MPDU GUI ==
  data: mpdu input; openGUIBoolean parameter boolean size=[1 1]
  events: trigger input FALLING_EDGE_EVENT
function mpduGUI(mpdu, openGUIBoolean)
%#codegen

coder.extrinsic('receivedMPDUGUI')

receivedMPDUGUI(mpdu, openGUIBoolean);

== matlab function project/802.11 Receiver/Detector/MPDU Decoder ==
  data: mpduCRC output; plcpCRC input; expLen input; actLen input; payload input; mpdu output Bus: BeaconMPDUType size=[1 1]
function [mpduCRC, mpdu] = mpduDec(plcpCRC, expLen, actLen, payload)
%#codegen

coder.extrinsic('warning')

persistent hCRC firstTime lastMPDU lastMpduCRC

% Frame check sequence (FCS)
if isempty(hCRC)
  hCRC = comm.CRCDetector([32 26 23 22 16 12 11 10 8 7 5 4 2 1 0], ...
    'InitialConditions', 1, ...
    'DirectMethod',      true, ...
    'FinalXOR',          1);
  firstTime = true;
  lastMPDU.Header = parseMPDUHeader(zeros(64,1), 1);
  lastMPDU.FrameBody = unknownMPDU();
  lastMpduCRC = true;  % CRC is not zero
end

% If the CRC for the header decodes correctly (i.e. CRC flag is 0) and the
% received MPDU payload length is greater than or equal to the expected
% length, then turn on the MPDU decoder
if ~plcpCRC && (expLen > 0) && (actLen >= expLen) && (expLen >= 32) ...
    && firstTime
  % Compute CRC based on IEEE Std 802.11(TM)-2007 section 7.1.3.7.
  frameCRC = payload(1:expLen);
  [frame, mpduCRC] = step(hCRC, frameCRC);
  
  [mpdu.Header, mpduHeaderLen] = parseMPDUHeader(frame, mpduCRC);
  
  if (mpduCRC == 1) || ((mpdu.Header.FrameCtrl.Type ~= 0) ...
      || (mpdu.Header.FrameCtrl.Subtype ~= 8))
    mpdu.FrameBody = unknownMPDU();
  else
    mpdu.FrameBody = parseBeaconMPDU(frame(mpduHeaderLen+1:end, 1), mpduCRC);
  end
  
  lastMPDU = mpdu;
  lastMpduCRC = mpduCRC;
  firstTime = false;
else
  mpdu = lastMPDU;
  mpduCRC = lastMpduCRC;
end
end

function [mpduHeader, len] = parseMPDUHeader(frame, mpduCRC)
% Based on IEEE Std 802.11-2007 chapter 7.

mpduHeader.FrameCtrl       = parseFrameControl(frame(1:16,1), mpduCRC);
mpduHeader.DurationID      = zeros(1,2,'uint8');
mpduHeader.Address1        = zeros(1,6,'uint8');
mpduHeader.Address2        = zeros(1,6,'uint8');
mpduHeader.Address3        = zeros(1,6,'uint8');
mpduHeader.SequenceControl = zeros(1,2,'uint8');
mpduHeader.Address4        = zeros(1,6,'uint8');
len = (2+6+6+6+2+6)*8 + 16;

if (mpduCRC == 0)
  p = 1;
  mpduHeader.FrameCtrl       = parseFrameControl(frame(p:p+15,1), mpduCRC);
  p = p+16;
  mpduHeader.DurationID      = bit2Octet(frame(p:p+15,1),2);
  p = p+16;
  mpduHeader.Address1        = bit2Octet(frame(p:p+47,1),6);
  p = p+48;

  isManagementFrame = (mpduHeader.FrameCtrl.Type == 0);
  isControlFrame = (mpduHeader.FrameCtrl.Type == 1);
  isDataFrame = (mpduHeader.FrameCtrl.Type == 2);
  isCTSFrame = isControlFrame && (mpduHeader.FrameCtrl.Subtype == 12);
  isACKFrame = isControlFrame && (mpduHeader.FrameCtrl.Subtype == 13);
  
  if ~(isCTSFrame || isACKFrame)
    mpduHeader.Address2        = bit2Octet(frame(p:p+47,1),6);
    p = p+48;
  end
  if isManagementFrame 
    mpduHeader.Address3        = bit2Octet(frame(p:p+47,1),6);
    p = p+48;
  end
  if ~isControlFrame
    mpduHeader.SequenceControl = bit2Octet(frame(p:p+15,1),2);
    p = p+16;
  end
  if isDataFrame
    mpduHeader.Address4        = bit2Octet(frame(p:p+47,1),6);
    p = p+48;
  end
  len = p-1;
end
end

function frameCtrl = parseFrameControl(fcBits, mpduCRC)
if (mpduCRC == 0)
  frameCtrl.ProtocolVersion = uint8(bi2de(fcBits(1:2,1)'));
  frameCtrl.Type            = uint8(bi2de(fcBits(3:4,1)'));
  frameCtrl.Subtype         = uint8(bi2de(fcBits(5:8,1)'));
  frameCtrl.ToDS            = uint8(bi2de(fcBits(9,1)'));
  frameCtrl.FromDS          = uint8(bi2de(fcBits(10,1)'));
  frameCtrl.MoreFragments   = uint8(bi2de(fcBits(11,1)'));
  frameCtrl.Retry           = uint8(bi2de(fcBits(12,1)'));
  frameCtrl.PowerManagement = uint8(bi2de(fcBits(13,1)'));
  frameCtrl.MoreData        = uint8(bi2de(fcBits(14,1)'));
  frameCtrl.ProtectedFrame  = uint8(bi2de(fcBits(15,1)'));
  frameCtrl.Order           = uint8(bi2de(fcBits(16,1)'));
else
  frameCtrl.ProtocolVersion = uint8(0);
  frameCtrl.Type            = uint8(0);
  frameCtrl.Subtype         = uint8(0);
  frameCtrl.ToDS            = uint8(0);
  frameCtrl.FromDS          = uint8(0);
  frameCtrl.MoreFragments   = uint8(0);
  frameCtrl.Retry           = uint8(0);
  frameCtrl.PowerManagement = uint8(0);
  frameCtrl.MoreData        = uint8(0);
  frameCtrl.ProtectedFrame  = uint8(0);
  frameCtrl.Order           = uint8(0);
end
end

function frameBody = parseBeaconMPDU(frame, mpduCRC)
if (mpduCRC == 0)
  bitCount = uint32(1);
  frameBody.TimeStamp      = bit2Octet(frame(bitCount:bitCount+63,1),8);
  bitCount = bitCount + 64;
  frameBody.BeaconInterval = bit2Octet(frame(bitCount:bitCount+15,1),2);
  bitCount = bitCount + 16;
  frameBody.Capability     = parseCapabilities(frame(81:96), mpduCRC);
  bitCount = bitCount + 16;
else
  frameBody.TimeStamp      = zeros(1,8,'uint8');
  frameBody.BeaconInterval = zeros(1,2,'uint8');
  frameBody.Capability     = parseCapabilities(frame(81:96), mpduCRC);
  bitCount = uint32(97);
end

frameLength = length(frame);

frameBody.NumInfoElements = uint8(0);
macElementStruct = struct('ID', uint8(255), ...
  'Length', uint8(0), ...
  'Value', zeros(1,257,'uint8'));
frameBody.InfoElements = repmat(macElementStruct, 1, 60);

if (mpduCRC == 0)
  while bitCount < frameLength
    frameBody.NumInfoElements = frameBody.NumInfoElements + 1;
    frameBody.InfoElements(frameBody.NumInfoElements).ID = ...
      bit2Octet(frame(bitCount:bitCount+7,1), 1);
    bitCount = bitCount + 8;
    elemLength = bit2Octet(frame(bitCount:bitCount+7,1), 1);
    frameBody.InfoElements(frameBody.NumInfoElements).Length = elemLength;
    bitCount = bitCount + 8;
    for p=1:elemLength
      frameBody.InfoElements(frameBody.NumInfoElements).Value(p) = ...
        bit2Octet(frame(bitCount:bitCount+7),1);
      bitCount = bitCount+8;
    end
  end
end
end

function capability = parseCapabilities(frame, mpduCRC)
if (mpduCRC == 0)
  capability.ESS                = frame(1,1);
  capability.IBSS               = frame(2,1);
  capability.CFPollable         = frame(3,1);
  capability.CFPollRequest      = frame(4,1);
  capability.Privacy            = frame(5,1);
  capability.ShortPreamble      = frame(6,1);
  capability.PBCC               = frame(7,1);
  capability.ChannelAgility     = frame(8,1);
  capability.SpectrumManagement = frame(9,1);
  capability.QoS                = frame(10,1);
  capability.ShortSlotTime      = frame(11,1);
  capability.APSD               = frame(12,1);
  capability.Reserved           = frame(13,1);
  capability.DSSOFDM            = frame(14,1);
  capability.DelayedBlockAck    = frame(15,1);
  capability.ImmediateBlockAck  = frame(16,1);
else
  capability.ESS                = false;
  capability.IBSS               = false;
  capability.CFPollable         = false;
  capability.CFPollRequest      = false;
  capability.Privacy            = false;
  capability.ShortPreamble      = false;
  capability.PBCC               = false;
  capability.ChannelAgility     = false;
  capability.SpectrumManagement = false;
  capability.QoS                = false;
  capability.ShortSlotTime      = false;
  capability.APSD               = false;
  capability.Reserved           = false;
  capability.DSSOFDM            = false;
  capability.DelayedBlockAck    = false;
  capability.ImmediateBlockAck  = false;
end
end

function frameBody = unknownMPDU()
frameBody.TimeStamp      = zeros(1,8,'uint8');
frameBody.BeaconInterval = zeros(1,2,'uint8');
frameBody.Capability     = parseCapabilities(zeros(16,1), 1);

frameBody.NumInfoElements = uint8(0);
macElementStruct = struct('ID', uint8(255), ...
  'Length', uint8(0), ...
  'Value', zeros(1,257,'uint8'));
frameBody.InfoElements = repmat(macElementStruct, 1, 60);
end

function octets = bit2Octet(bits,numOctets)
octets = zeros(1, numOctets, 'uint8');
for p=1:numOctets
  octets(1,p) = (bits((p-1)*8+1:p*8)')*2.^(0:7)';
end
end

== matlab function project/802.11 Receiver/Detector/Packet Parser ==
  data: plcpLength output; plcp output size=[p80211.PLCPLength - length(p80211.SYNC) + length(p80211.ScramblerPolynomial) 1]; payloadLength output; bits input; plcpIdx input size=2; payloadIdx input size=2; p80211 parameter; payload output size=[1024 1]
function [plcpLength, plcp, payloadLength, payload] = ...
  packetParser(bits, plcpIdx, payloadIdx, p80211)

%#codegen

persistent plcpCount payloadCount plcpBuffer payloadBuffer

if isempty(plcpCount)
  plcpCount = uint16(1);
  payloadCount = uint16(1);
  % 8 extra bits for syncronizing descrambler
  plcpBuffer = false(p80211.PLCPLength - length(p80211.SYNC) ...
    + length(p80211.ScramblerPolynomial), 1);
  payloadBuffer = false(1024, 1);
end

% First fill PLCP buffer
% Since plcpIdx will be [2 1] if there is no data for PLCP and
% plcpCounter is uint16, we first need to add with plcpCounter to avoid
% negative numbers.
startIdx = plcpCount;
endIdx = (plcpCount+plcpIdx(2,1))-plcpIdx(1,1);
plcpBuffer(startIdx:endIdx) = bits(plcpIdx(1,1):plcpIdx(2,1));
plcpCount = plcpCount + (1 + endIdx) - startIdx;
plcpLength = plcpCount - 1;

% Fill the payload buffer
startIdx = payloadCount;
endIdx = (payloadCount+payloadIdx(2,1))-payloadIdx(1,1);
payloadBuffer(startIdx:endIdx) = bits(payloadIdx(1,1):payloadIdx(2,1));
payloadCount = payloadCount + (1 + endIdx) - startIdx;
payloadLength = payloadCount - 1; 

plcp = plcpBuffer;
payload = payloadBuffer;

== matlab function project/802.11 Receiver/Receiver Controller/Rx Controller ==
  data: preambleIdx input; corrVal input; startRx output; plcpIdx output; payloadIdx output; headerCRC input boolean size=[1 1]; payloadLength input size=1; p80211 parameter; syncDelay output
function [startRx, plcpIdx, payloadIdx, syncDelay] = ...
  rxCtrl(preambleIdx, corrVal, headerCRC, payloadLength, p80211)
%#codegen

persistent rxOn controllerState plcpCount payloadCount lastSyncDelay

% State Enums
SearchPLCP = 0;
WaitForSFD = 1;
GetPLCP    = 2;
DecodePLCP = 3;
GetPayload = 4;
WindDownRx = 5;

if isempty(rxOn)
  % Initialize receiver controller
  rxOn = false;
  controllerState = SearchPLCP;
  plcpCount    = 0;
  payloadCount = 0;
  lastSyncDelay = 0;
end

plcpIdx    = [2 1]; % No samples for PLCP
payloadIdx = [2 1]; % No samples for payload


switch controllerState
  case SearchPLCP
    if ~isempty(preambleIdx)
      [~,idx] = max(corrVal(preambleIdx));
      prbIdx = preambleIdx(idx);
      % Synchronize to the end of the SYNC. Get 8 (scrambler length) extra
      % bits to initialize DPSK demodulator and scrambler
      scramblerLen = length(p80211.ScramblerPolynomial);
      lastSyncDelay = p80211.SamplesPerChannelFrame - (prbIdx ...
        - scramblerLen*p80211.SpreadingRate*p80211.SamplesPerChip); 
      plcpCount = p80211.NumSYNCSamples ...
        - scramblerLen*p80211.SpreadingRate*p80211.SamplesPerChip;
      rxOn = true;
      
      controllerState = WaitForSFD;
    end
  case WaitForSFD
      rxOn = true;
      controllerState = GetPLCP;
  case GetPLCP
    % In this state we recevie both SFD, which is part of PLCP preamble,
    % and the PLCP header
    
    plcpCount = plcpCount + p80211.SamplesPerChannelFrame;
    
    if (plcpCount >= p80211.NumPLCPSamples)
      payloadCount = plcpCount - p80211.NumPLCPSamples;
      headerEndIdx = p80211.BitsPerChannelFrame - (payloadCount / ...
        (p80211.SamplesPerChip*p80211.SpreadingRate));
      plcpIdx = [1 headerEndIdx];
      payloadIdx = [plcpIdx(2)+1 p80211.BitsPerChannelFrame];

      controllerState = DecodePLCP;
    else
      plcpIdx = [1 p80211.BitsPerChannelFrame];
    end
  case DecodePLCP
    payloadCount = payloadCount + p80211.SamplesPerChannelFrame;
    
    payloadIdx = [1 p80211.BitsPerChannelFrame];
    
    if (headerCRC == 0)
      controllerState = GetPayload;
    else
      % Abbort reception
      rxOn = false;
      lastSyncDelay = 0;
      payloadCount = 0;
      controllerState = SearchPLCP;
    end
  case GetPayload
    payloadCount = payloadCount + p80211.SamplesPerChannelFrame;
    
    if payloadCount >= payloadLength
      controllerState = WindDownRx;
    end
    
    payloadIdx = [1 p80211.BitsPerChannelFrame];
  case WindDownRx
    rxOn = false;
    lastSyncDelay = 0;
    payloadCount = 0;
    controllerState = SearchPLCP;
end

startRx = rxOn;
syncDelay = lastSyncDelay;

== matlab function project/802.11 Transmitter/MAC Sublayer/Transmitter Controller ==
  settings: updateMethod=DISCRETE  sampleTime=p80211.MaximumPPDULength/p80211.SymbolRate
  data: payload output uint8 size=[p80211.MaximumMPDULength 1]; startTx output boolean; p80211 parameter
function [payload, startTx] = txCtrl(p80211)
%#codegen

persistent xmtState txOn mpduCount TSF

% States
Idle     = 0;
Transmit = 1;

% Initialize transmitter
if isempty(xmtState)
  TSF = zeros(2,1,'uint32');
  xmtState = Idle;
  txOn = false;
  mpduCount = p80211.BeaconInterval-1;
end

% Init payload buffer
[mpduHeader, mpduBody] = getBeaconMPDU(TSF, p80211);
payload = serializeMPDUData(mpduHeader, mpduBody);

% Update counter
mpduCount = mpduCount + 1;

% State machine
switch xmtState
  case Idle,
    if (mpduCount >= p80211.BeaconInterval)
      mpduCount = 0;
      [mpduHeader, mpduBody] = getBeaconMPDU(TSF, p80211);
      payload = serializeMPDUData(mpduHeader, mpduBody);
      txOn = true;
      xmtState = Transmit;
    end
  case Transmit,
      txOn = false;
      xmtState = Idle;
end

% Update TSF
oldTSF1 = TSF(1);
% Since bit rate is 1 Mbps, every bit is one microsecond.  Also, the
% transmitter works every (p80211.MaximumPPDULength = 1024) TU.
TSF(1) = TSF(1) + uint32(p80211.MaximumPPDULength); 
if oldTSF1 > TSF(1)
  TSF(2) = TSF(2) + 1;
end

% Update outputs
startTx = txOn;
end
